simulink model "generic_uservehicle"  (Simulink 7.5)
settings: Solver=ode45  StartTime=0.0  StopTime=inf  RelTol=1e-3
libraries: simulink x6, CarMaker4SL x1
(part 1 of 3)
settings Model: Creator=fh  LastModifiedBy=ml  ExtModeAutoUpdateStatusClock=off
settings DataIOCC: SignalLoggingName=sigsOut
settings OptimizationCC: BooleanDataType=off  InitFltsAndDblsToZero=on
settings DebuggingCC: SaveWithParameterizedLinksMsg=none  SignalResolutionControl=TryResolveAllWithWarning  SolverPrmCheckMsg=none  MultiTaskDSMMsg=warning  MultiTaskCondExecSysMsg=none
settings HardwareCC: TargetUnknown=on
settings RTWCC: IncludeERTFirstTime=on
settings CodeAppCC: MaxIdLength=63
settings GRTTargetCC: TargetFcnLib=ansi_tfl_tmw.mat

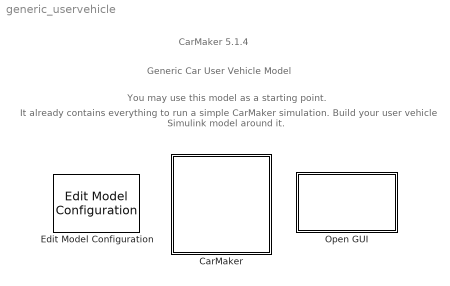
== system generic_uservehicle ==
  note: Generic Car User Vehicle Model
  note: CarMaker 5.1.4
  note: You may use this model as a starting point.
  note: It already contains everything to run a simple CarMaker simulation.
      | Build your user vehicle Simulink model around it.
  CarMaker : Subsystem  TreatAsAtomicUnit=on
      mask Display: image(imread('CarMaker4SLss.bmp'));
  Edit Model Configuration : CarMaker4SL/Edit Model Configuration
  Open GUI : Subsystem  LoadFcn=if ~length(which('cmcmd')), cmenv; end
      settings: OpenFcn=cmblockmagic('gui_fix_display'); CM_Simulink
      mask Display: image(imread('CarMakerGUI.bmp'));

== system generic_uservehicle/CarMaker ==
  CM_FIRST : Subsystem
  CM_LAST : Subsystem
  DrivMan : Subsystem
  Ground : Ground
  Terminator : Terminator
  Vehicle : Subsystem
  VehicleControl : Subsystem
  wires:
  DrivMan/2(DrivMan.Out) -> VehicleControl/2(DrivMan.In)
  DrivMan/1(Sync_Out) -> VehicleControl/1(Sync_In)
  CM_FIRST/2(Env.Misc) -> DrivMan/2(Env.Misc)
  CM_FIRST/1(Sync_Out) -> DrivMan/1(Sync_In)
  CM_LAST/1(Sync_Out) -> Terminator/1
  Ground/1 -> CM_FIRST/1(Sync_In)
  Vehicle/1(Sync_Out) -> CM_LAST/1(Sync_In)
  VehicleControl/1(Sync_Out) -> Vehicle/1(Sync_In)
  VehicleControl/3(VhclCtrl.Steering) -> Vehicle/3(VhclCtrl.Steering)
  VehicleControl/4(Vhcl.Wheel.In) -> Vehicle/4(Vhcl.Wheel.In)
  VehicleControl/5(Vhcl.Misc) -> Vehicle/5(Vhcl.Misc)
  VehicleControl/6(VhclCtrl.Brake) -> Vehicle/6(VhclCtrl.Brake)
  VehicleControl/7(VhclCtrl.PT) -> Vehicle/7(VhclCtrl.PT)
  VehicleControl/2(Vhcl.Model.Source) -> Vehicle/2(Vhcl.Model.Source)

== system generic_uservehicle/Open GUI ==
  S-Function : S-Function  FunctionName=cm_gui  EnableBusSupport=off

== system generic_uservehicle/CarMaker/CM_FIRST ==
  Sync_In : Inport  OutDataType=sfix(16)  OutScaling=2^0
  Bus Creator1 : BusCreator  Inputs=9
  Demux : Demux  Outputs=9
  Environment : S-Function  FunctionName=CM_Sfun  Parameters='Environment'  EnableBusSupport=off
  IoIn : S-Function  FunctionName=CM_Sfun  Parameters='IoIn'  EnableBusSupport=off
  Sync_Out : Outport  OutDataType=sfix(16)  OutScaling=2^0
  Env.Misc : Outport  Port=2  OutDataType=sfix(16)  OutScaling=2^0
  wires:
  Demux/9 -> Bus Creator1/9  "Env WindVel_tot z"
  Demux/8 -> Bus Creator1/8  "Env WindVel_tot y"
  Demux/7 -> Bus Creator1/7  "Env WindVel_tot x"
  Demux/6 -> Bus Creator1/6  "Env SolarRadiation"
  Demux/5 -> Bus Creator1/5  "Env Time"
  Sync_In/1 -> IoIn/1
  IoIn/1 -> Environment/1
  Environment/1 -> Sync_Out/1
  Demux/1 -> Bus Creator1/1  "Env Temperature"
  Demux/2 -> Bus Creator1/2  "Env AirDensity"
  Demux/3 -> Bus Creator1/3  "Env AirPressure"
  Demux/4 -> Bus Creator1/4  "Env AirHumidity"
  Environment/2 -> Demux/1
  Bus Creator1/1 -> Env.Misc/1

== system generic_uservehicle/CarMaker/CM_LAST ==
  Sync_In : Inport  OutDataType=sfix(16)  OutScaling=2^0
  CM_User : S-Function  FunctionName=CM_Sfun  Parameters='CM_User'  EnableBusSupport=off
  IoOut : S-Function  FunctionName=CM_Sfun  Parameters='IoOut'  EnableBusSupport=off
  Sync_Out : Outport  OutDataType=sfix(16)  OutScaling=2^0
  wires:
  IoOut/1 -> Sync_Out/1
  CM_User/1 -> IoOut/1
  Sync_In/1 -> CM_User/1

== system generic_uservehicle/CarMaker/DrivMan ==
  note: There's rarely a reason to override DrivMan signals.
      | Use the VehicleControl interface for this purpose.
  Sync_In : Inport  OutDataType=sfix(16)  OutScaling=2^0
  Env.Misc : Inport  Port=2  OutDataType=sfix(16)  OutScaling=2^0
  BusCreator : BusCreator  Inputs=17
  Demux : Demux  Outputs=17
  DrivMan : S-Function  FunctionName=CM_Sfun  Parameters='DrivMan'  EnableBusSupport=off
  Sync_Out : Outport  OutDataType=sfix(16)  OutScaling=2^0
  DrivMan.Out : Outport  Port=2  OutDataType=sfix(16)  OutScaling=2^0
  wires:
  Demux/17 -> BusCreator/17  "DrivMan Steering Trq"
  Demux/16 -> BusCreator/16  "DrivMan Steering AngAcc"
  Demux/15 -> BusCreator/15  "DrivMan Steering AngVel"
  Demux/14 -> BusCreator/14  "DrivMan Steering Ang"
  Demux/13 -> BusCreator/13  "DrivMan Gas"
  Demux/12 -> BusCreator/12  "DrivMan Clutch"
  Demux/11 -> BusCreator/11  "DrivMan BrakePark"
  Demux/10 -> BusCreator/10  "DrivMan Brake"
  Demux/9 -> BusCreator/9  "DrivMan GearNo"
  Demux/8 -> BusCreator/8  "DrivMan SelectorCtrl"
  Demux/7 -> BusCreator/7  "DrivMan UserSignal4"
  Demux/6 -> BusCreator/6  "DrivMan UserSignal3"
  Demux/5 -> BusCreator/5  "DrivMan UserSignal2"
  Demux/4 -> BusCreator/4  "DrivMan UserSignal1"
  Demux/3 -> BusCreator/3  "DrivMan UserSignal0"
  Demux/2 -> BusCreator/2  "DrivMan Key"
  Demux/1 -> BusCreator/1  "DrivMan SST"
  Env.Misc/1 -> DrivMan/2
  Sync_In/1 -> DrivMan/1
  DrivMan/1 -> Sync_Out/1
  BusCreator/1 -> DrivMan.Out/1
  DrivMan/2 -> Demux/1

== system generic_uservehicle/CarMaker/Vehicle ==
  note: The enabled subsystems allow for simultaneous availability of more than one vehicle.
      | Which one to use will be determined by the vehicle data set of the testrun.
      | If this functionality is not needed, you may simplify your model by using
      | the relevant subsystem of the three as a drop-in replacement for the
      | 'Vehicle' subsystem you're currently looking at, as is done in most of the
      | CarMaker for Simulink example models.
      |
      | PLEASE NOTE: In CarMaker/HIL-ds100x vehicle switching depending on
      | the vehicle data set is not available. To run the user vehicle, the command
      | line option -disablevehicle in the Model Configuration block is required.
  Sync_In : Inport  OutDataType=sfix(16)  OutScaling=2^0
  Vhcl.Model.Source : Inport  Port=2  OutDataType=sfix(16)  OutScaling=2^0
  VhclCtrl.Steering : Inport  Port=3  OutDataType=sfix(16)  OutScaling=2^0
  Vhcl.Wheel.In : Inport  Port=4  OutDataType=sfix(16)  OutScaling=2^0
  Vhcl.Misc : Inport  Port=5  OutDataType=sfix(16)  OutScaling=2^0
  VhclCtrl.Brake : Inport  Port=6  OutDataType=sfix(16)  OutScaling=2^0
  VhclCtrl.PT : Inport  Port=7  OutDataType=sfix(16)  OutScaling=2^0
  IPG Vehicle : Subsystem  TreatAsAtomicUnit=on
  Multiport Switch : MultiPortSwitch  zeroidx=off  InputSameDT=on
  User Vehicle (CM4SL) : Subsystem  TreatAsAtomicUnit=on
  User Vehicle (ModelMgr) : Subsystem  TreatAsAtomicUnit=on
  VehicleSource_BuiltIn : simulink/Logic and Bit Operations/Compare To Constant  SystemSampleTime=-1  relop===  const=1  LogicOutDataTypeMode=boolean  ZeroCross=off
  VehicleSource_CM4SL : simulink/Logic and Bit Operations/Compare To Constant  SystemSampleTime=-1  relop===  const=3  LogicOutDataTypeMode=boolean  ZeroCross=off
  VehicleSource_ModelMgr : simulink/Logic and Bit Operations/Compare To Constant  SystemSampleTime=-1  relop===  const=2  LogicOutDataTypeMode=boolean  ZeroCross=off
  Sync_Out : Outport  OutDataType=sfix(16)  OutScaling=2^0
  wires:
  VhclCtrl.Steering/1 -> IPG Vehicle/3(VhclCtrl.Steering), User Vehicle (ModelMgr)/3(VhclCtrl.Steering), User Vehicle (CM4SL)/3(VhclCtrl.Steering)
  Vhcl.Wheel.In/1 -> IPG Vehicle/4(Vhcl.Wheel.In), User Vehicle (ModelMgr)/4(Vhcl.Wheel.In), User Vehicle (CM4SL)/4(Vhcl.Wheel.In)
  Vhcl.Misc/1 -> IPG Vehicle/5(Vhcl.Misc), User Vehicle (ModelMgr)/5(Vhcl.Misc), User Vehicle (CM4SL)/5(Vhcl.Misc)
  VehicleSource_BuiltIn/1 -> IPG Vehicle/Enable
  VhclCtrl.Brake/1 -> IPG Vehicle/6(VhclCtrl.Brake), User Vehicle (ModelMgr)/6(VhclCtrl.Brake), User Vehicle (CM4SL)/6(VhclCtrl.Brake)
  VhclCtrl.PT/1 -> IPG Vehicle/7(VhclCtrl.PT), User Vehicle (ModelMgr)/7(VhclCtrl.PT), User Vehicle (CM4SL)/7(VhclCtrl.PT)
  Sync_In/1 -> IPG Vehicle/1(Sync_In), User Vehicle (ModelMgr)/1(Sync_In), User Vehicle (CM4SL)/1(Sync_In)
  Vhcl.Model.Source/1 -> VehicleSource_ModelMgr/1, VehicleSource_BuiltIn/1, Multiport Switch/1, IPG Vehicle/2(Vhcl.Model.Source), User Vehicle (ModelMgr)/2(Vhcl.Model.Source), User Vehicle (CM4SL)/2(Vhcl.Model.Source), VehicleSource_CM4SL/1
  VehicleSource_CM4SL/1 -> User Vehicle (CM4SL)/Enable
  VehicleSource_ModelMgr/1 -> User Vehicle (ModelMgr)/Enable
  IPG Vehicle/1(Sync_Out) -> Multiport Switch/2
  User Vehicle (ModelMgr)/1(Sync_Out) -> Multiport Switch/3
  User Vehicle (CM4SL)/1(Sync_Out) -> Multiport Switch/4
  Multiport Switch/1 -> Sync_Out/1

== system generic_uservehicle/CarMaker/VehicleControl ==
  note: <Your model here>
  note: When implementing a vehicle control model,
      | be sure to add '-disablevehiclecontrol' to the command line arguments
      | in the CarMaker Model Configuration block.
      | Otherwise your model will possibly not see the original DrivMan signals
      | on its inputs, but those of a currently activated C-coded vehicle control model instead.
  Sync_In : Inport  OutDataType=sfix(16)  OutScaling=2^0
  DrivMan.In : Inport  Port=2  OutDataType=sfix(16)  OutScaling=2^0
  Bus Creator2 : BusCreator  Inputs=2
  CreateBus Vhcl.Misc : Subsystem
  CreateBus Vhcl.Wheel.In : Subsystem
  CreateBus VhclCtrl : Subsystem
  CreateBus VhclCtrl.PT : Subsystem
  CreateBus VhclCtrl.Steering : Subsystem
  Demux2 : Demux  Outputs=2
  VehicleControl : S-Function  FunctionName=CM_Sfun  Parameters='VehicleControl'  EnableBusSupport=off
  VehicleControlUpd : S-Function  FunctionName=CM_Sfun  Parameters='VehicleControlUpd'  EnableBusSupport=off
  Sync_Out : Outport  OutDataType=sfix(16)  OutScaling=2^0
  Vhcl.Model.Source : Outport  Port=2  OutDataType=sfix(16)  OutScaling=2^0
  VhclCtrl.Steering : Outport  Port=3  OutDataType=sfix(16)  OutScaling=2^0
  Vhcl.Wheel.In : Outport  Port=4  OutDataType=sfix(16)  OutScaling=2^0
  Vhcl.Misc : Outport  Port=5  OutDataType=sfix(16)  OutScaling=2^0
  VhclCtrl.Brake : Outport  Port=6  OutDataType=sfix(16)  OutScaling=2^0
  VhclCtrl.PT : Outport  Port=7  OutDataType=sfix(16)  OutScaling=2^0
  wires:
  CreateBus VhclCtrl/1(Out) -> VehicleControlUpd/2
  VehicleControl/2 -> CreateBus VhclCtrl/1(In)
  VehicleControlUpd/2 -> Vhcl.Model.Source/1
  VehicleControlUpd/4 -> CreateBus Vhcl.Wheel.In/1(In1)
  VehicleControlUpd/5 -> CreateBus Vhcl.Misc/1(In1)
  VehicleControlUpd/6 -> Demux2/1
  VehicleControlUpd/7 -> CreateBus VhclCtrl.PT/1(In1)
  VehicleControlUpd/3 -> CreateBus VhclCtrl.Steering/1(In1)
  CreateBus Vhcl.Misc/1(Out1) -> Vhcl.Misc/1
  CreateBus Vhcl.Wheel.In/1(Out1) -> Vhcl.Wheel.In/1
  DrivMan.In/1 -> VehicleControl/2
  VehicleControl/1 -> VehicleControlUpd/1
  Sync_In/1 -> VehicleControl/1
  CreateBus VhclCtrl.PT/1(Out1) -> VhclCtrl.PT/1
  Bus Creator2/1 -> VhclCtrl.Brake/1
  CreateBus VhclCtrl.Steering/1(Out1) -> VhclCtrl.Steering/1
  VehicleControlUpd/1 -> Sync_Out/1
  Demux2/2 -> Bus Creator2/2  "VhclCtrl BrakePark"
  Demux2/1 -> Bus Creator2/1  "VhclCtrl Brake"

== system generic_uservehicle/CarMaker/Vehicle/IPG Vehicle ==
  Sync_In : Inport  OutDataType=sfix(16)  OutScaling=2^0
  Vhcl.Model.Source : Inport  Port=2  OutDataType=sfix(16)  OutScaling=2^0
  VhclCtrl.Steering : Inport  Port=3  OutDataType=sfix(16)  OutScaling=2^0
  Vhcl.Wheel.In : Inport  Port=4  OutDataType=sfix(16)  OutScaling=2^0
  Vhcl.Misc : Inport  Port=5  OutDataType=sfix(16)  OutScaling=2^0
  VhclCtrl.Brake : Inport  Port=6  OutDataType=sfix(16)  OutScaling=2^0
  VhclCtrl.PT : Inport  Port=7  OutDataType=sfix(16)  OutScaling=2^0
  Enable : EnablePort
  Brake : Subsystem
  CarAndTrailer : Subsystem
  PowerTrain : Subsystem
  Stop Simulation : Stop
  VehicleSource_BuiltIn : simulink/Logic and Bit Operations/Compare To Constant  SystemSampleTime=-1  relop=~=  const=1  LogicOutDataTypeMode=boolean  ZeroCross=off
  Sync_Out : Outport  OutDataType=sfix(16)  OutScaling=2^0
  wires:
  VhclCtrl.PT/1 -> PowerTrain/3(VhclCtrl.PT)
  CarAndTrailer/1(Sync_Out) -> Brake/1(Sync_In)
  CarAndTrailer/2(Brake.IF.In) -> Brake/2(Brake.IF.In)
  VhclCtrl.Brake/1 -> Brake/3(VhclCtrl.Brake)
  PowerTrain/1(Sync_Out) -> Sync_Out/1
  Vhcl.Misc/1 -> CarAndTrailer/4(Vhcl.Misc)
  Vhcl.Wheel.In/1 -> CarAndTrailer/3(Vhcl.Wheel.In)
  VhclCtrl.Steering/1 -> CarAndTrailer/2(VhclCtrl.Steering)
  Sync_In/1 -> CarAndTrailer/1(Sync_In)
  Vhcl.Model.Source/1 -> VehicleSource_BuiltIn/1
  VehicleSource_BuiltIn/1 -> Stop Simulation/1
  Brake/1(Sync_Out) -> PowerTrain/1(Sync_In)
  Brake/2(Vhcl.Wheel.PT) -> PowerTrain/2(Vhcl.Wheel.PT)

== system generic_uservehicle/CarMaker/Vehicle/User Vehicle (CM4SL) ==
  Sync_In : Inport  OutDataType=sfix(16)  OutScaling=2^0
  Vhcl.Model.Source : Inport  Port=2  OutDataType=sfix(16)  OutScaling=2^0
  VhclCtrl.Steering : Inport  Port=3  OutDataType=sfix(16)  OutScaling=2^0
  Vhcl.Wheel.In : Inport  Port=4  OutDataType=sfix(16)  OutScaling=2^0
  Vhcl.Misc : Inport  Port=5  OutDataType=sfix(16)  OutScaling=2^0
  VhclCtrl.Brake : Inport  Port=6  OutDataType=sfix(16)  OutScaling=2^0
  VhclCtrl.PT : Inport  Port=7  OutDataType=sfix(16)  OutScaling=2^0
  Enable : EnablePort
  Brake : Subsystem
  CarAndTrailer : Subsystem
  PowerTrain : Subsystem
  Stop Simulation : Stop
  VehicleSource_CM4SL : simulink/Logic and Bit Operations/Compare To Constant  SystemSampleTime=-1  relop=~=  const=3  LogicOutDataTypeMode=boolean  ZeroCross=off
  Sync_Out : Outport  OutDataType=sfix(16)  OutScaling=2^0
  wires:
  VehicleSource_CM4SL/1 -> Stop Simulation/1
  Sync_In/1 -> CarAndTrailer/1(Sync_In)
  VhclCtrl.Steering/1 -> CarAndTrailer/2(VhclCtrl.Steering)
  Vhcl.Wheel.In/1 -> CarAndTrailer/3(Vhcl.Wheel.In)
  Vhcl.Misc/1 -> CarAndTrailer/4(Vhcl.Misc)
  PowerTrain/1(Sync_Out) -> Sync_Out/1
  VhclCtrl.Brake/1 -> Brake/3(VhclCtrl.Brake)
  CarAndTrailer/2(Brake.IF.In) -> Brake/2(Brake.IF.In)
  CarAndTrailer/1(Sync_Out) -> Brake/1(Sync_In)
  VhclCtrl.PT/1 -> PowerTrain/3(VhclCtrl.PT)
  Vhcl.Model.Source/1 -> VehicleSource_CM4SL/1
  Brake/1(Sync_Out) -> PowerTrain/1(Sync_In)
  Brake/2(Vhcl.Wheel.PT) -> PowerTrain/2(Vhcl.Wheel.PT)

== system generic_uservehicle/CarMaker/Vehicle/User Vehicle (ModelMgr) ==
  Sync_In : Inport  OutDataType=sfix(16)  OutScaling=2^0
  Vhcl.Model.Source : Inport  Port=2  OutDataType=sfix(16)  OutScaling=2^0
  VhclCtrl.Steering : Inport  Port=3  OutDataType=sfix(16)  OutScaling=2^0
  Vhcl.Wheel.In : Inport  Port=4  OutDataType=sfix(16)  OutScaling=2^0
  Vhcl.Misc : Inport  Port=5  OutDataType=sfix(16)  OutScaling=2^0
  VhclCtrl.Brake : Inport  Port=6  OutDataType=sfix(16)  OutScaling=2^0
  VhclCtrl.PT : Inport  Port=7  OutDataType=sfix(16)  OutScaling=2^0
  Enable : EnablePort
  Brake : Subsystem
  CarAndTrailer : Subsystem
  PowerTrain : Subsystem
  Stop Simulation : Stop
  VehicleSource_ModelMgr : simulink/Logic and Bit Operations/Compare To Constant  SystemSampleTime=-1  relop=~=  const=2  LogicOutDataTypeMode=boolean  ZeroCross=off
  Sync_Out : Outport  OutDataType=sfix(16)  OutScaling=2^0
  wires:
  Vhcl.Model.Source/1 -> VehicleSource_ModelMgr/1
  Sync_In/1 -> CarAndTrailer/1(Sync_In)
  VhclCtrl.Brake/1 -> Brake/3(VhclCtrl.Brake)
  VhclCtrl.PT/1 -> PowerTrain/3(VhclCtrl.PT)
  PowerTrain/1(Sync_Out) -> Sync_Out/1
  CarAndTrailer/1(Sync_Out) -> Brake/1(Sync_In)
  CarAndTrailer/2(Brake.IF.In) -> Brake/2(Brake.IF.In)
  Vhcl.Misc/1 -> CarAndTrailer/4(Vhcl.Misc)
  Vhcl.Wheel.In/1 -> CarAndTrailer/3(Vhcl.Wheel.In)
  VhclCtrl.Steering/1 -> CarAndTrailer/2(VhclCtrl.Steering)
  VehicleSource_ModelMgr/1 -> Stop Simulation/1
  Brake/1(Sync_Out) -> PowerTrain/1(Sync_In)
  Brake/2(Vhcl.Wheel.PT) -> PowerTrain/2(Vhcl.Wheel.PT)

== system generic_uservehicle/CarMaker/VehicleControl/CreateBus Vhcl.Misc ==
  In1 : Inport  OutDataType=sfix(16)  OutScaling=2^0
  Bus Creator5 : BusCreator  Inputs=11
  Demux5 : Demux  Outputs=11
  Out1 : Outport  OutDataType=sfix(16)  OutScaling=2^0
  wires:
  Demux5/11 -> Bus Creator5/11  "Vhcl Wind_vel_0 z"
  Demux5/10 -> Bus Creator5/10  "Vhcl Wind_vel_0 y"
  Demux5/9 -> Bus Creator5/9  "Vhcl Wind_vel_0 x"
  Demux5/8 -> Bus Creator5/8  "Vhcl DL2BdyEng y"
  Demux5/7 -> Bus Creator5/7  "Vhcl DL2BdyEng x"
  Demux5/6 -> Bus Creator5/6  "Vhcl TrqDL2Bdy1B z"
  Demux5/5 -> Bus Creator5/5  "Vhcl TrqDL2Bdy1B y"
  Demux5/4 -> Bus Creator5/4  "Vhcl TrqDL2Bdy1B x"
  Demux5/3 -> Bus Creator5/3  "Vhcl Trq_DL2Bdy1 z"
  In1/1 -> Demux5/1
  Bus Creator5/1 -> Out1/1
  Demux5/2 -> Bus Creator5/2  "Vhcl Trq_DL2Bdy1 y"
  Demux5/1 -> Bus Creator5/1  "Vhcl Trq_DL2Bdy1 x"

== system generic_uservehicle/CarMaker/VehicleControl/CreateBus Vhcl.Wheel.In ==
  In1 : Inport  OutDataType=sfix(16)  OutScaling=2^0
  Bus Creator1 : BusCreator  Inputs=12
  Demux1 : Demux  Outputs=12
  Out1 : Outport  OutDataType=sfix(16)  OutScaling=2^0
  wires:
  Demux1/12 -> Bus Creator1/12  "Vhcl Wheel RR rotv"
  Demux1/11 -> Bus Creator1/11  "Vhcl Wheel RR Trq_DL2WC"
  Demux1/10 -> Bus Creator1/10  "Vhcl Wheel RR Trq_B2WC"
  Demux1/9 -> Bus Creator1/9  "Vhcl Wheel RL rotv"
  Demux1/8 -> Bus Creator1/8  "Vhcl Wheel RL Trq_DL2WC"
  Demux1/7 -> Bus Creator1/7  "Vhcl Wheel RL Trq_B2WC"
  Demux1/6 -> Bus Creator1/6  "Vhcl Wheel FR rotv"
  Demux1/5 -> Bus Creator1/5  "Vhcl Wheel FR Trq_DL2WC"
  Demux1/4 -> Bus Creator1/4  "Vhcl Wheel FR Trq_B2WC"
  Demux1/3 -> Bus Creator1/3  "Vhcl Wheel FL rotv"
  In1/1 -> Demux1/1
  Bus Creator1/1 -> Out1/1
  Demux1/2 -> Bus Creator1/2  "Vhcl Wheel FL Trq_DL2WC"
  Demux1/1 -> Bus Creator1/1  "Vhcl Wheel FL Trq_B2WC"

== system generic_uservehicle/CarMaker/VehicleControl/CreateBus VhclCtrl ==
  In : Inport
  BusCreator : BusCreator  Inputs=29
  Demux : Demux  Outputs=29
  Out : Outport
  wires:
  In/1 -> Demux/1
  BusCreator/1 -> Out/1
  Demux/1 -> BusCreator/1  "VhclCtrl SST"
  Demux/2 -> BusCreator/2  "VhclCtrl Key"
  Demux/3 -> BusCreator/3  "VhclCtrl UserSignal0"
  Demux/4 -> BusCreator/4  "VhclCtrl UserSignal1"
  Demux/5 -> BusCreator/5  "VhclCtrl UserSignal2"
  Demux/6 -> BusCreator/6  "VhclCtrl UserSignal3"
  Demux/7 -> BusCreator/7  "VhclCtrl UserSignal4"
  Demux/8 -> BusCreator/8  "VhclCtrl GearNo"
  Demux/9 -> BusCreator/9  "VhclCtrl SelectorCtrl"
  Demux/10 -> BusCreator/10  "VhclCtrl Brake"
  Demux/11 -> BusCreator/11  "VhclCtrl BrakePark"
  Demux/12 -> BusCreator/12  "VhclCtrl Clutch"
  Demux/13 -> BusCreator/13  "VhclCtrl Gas"
  Demux/14 -> BusCreator/14  "VhclCtrl Steering Ang"
  Demux/15 -> BusCreator/15  "VhclCtrl Steering AngVel"
  Demux/16 -> BusCreator/16  "VhclCtrl Steering AngAcc"
  Demux/17 -> BusCreator/17  "VhclCtrl Steering Trq"
  Demux/18 -> BusCreator/18  "VhclCtrl Lights LowBeam"
  Demux/19 -> BusCreator/19  "VhclCtrl Lights HighBeam"
  Demux/20 -> BusCreator/20  "VhclCtrl Lights Daytime"
  Demux/21 -> BusCreator/21  "VhclCtrl Lights ParkL"
  Demux/22 -> BusCreator/22  "VhclCtrl Lights ParkR"
  Demux/23 -> BusCreator/23  "VhclCtrl Lights IndL"
  Demux/24 -> BusCreator/24  "VhclCtrl Lights IndR"
  Demux/25 -> BusCreator/25  "VhclCtrl Lights FogFrontL"
  Demux/26 -> BusCreator/26  "VhclCtrl Lights FogFrontR"
  Demux/27 -> BusCreator/27  "VhclCtrl Lights FogRear"
  Demux/28 -> BusCreator/28  "VhclCtrl Lights Brake"
  Demux/29 -> BusCreator/29  "VhclCtrl Lights Reverse"

== system generic_uservehicle/CarMaker/VehicleControl/CreateBus VhclCtrl.PT ==
  In1 : Inport
  BusCreator : BusCreator  Inputs=11
  Demux : Demux  Outputs=11
  Out1 : Outport
  wires:
  In1/1 -> Demux/1
  BusCreator/1 -> Out1/1
  Demux/1 -> BusCreator/1  "VhclCtrl SST"
  Demux/2 -> BusCreator/2  "VhclCtrl Key"
  Demux/3 -> BusCreator/3  "VhclCtrl UserSignal0"
  Demux/4 -> BusCreator/4  "VhclCtrl UserSignal1"
  Demux/5 -> BusCreator/5  "VhclCtrl UserSignal2"
  Demux/6 -> BusCreator/6  "VhclCtrl UserSignal3"
  Demux/7 -> BusCreator/7  "VhclCtrl UserSignal4"
  Demux/8 -> BusCreator/8  "VhclCtrl GearNo"
  Demux/9 -> BusCreator/9  "VhclCtrl SelectorCtrl"
  Demux/10 -> BusCreator/10  "VhclCtrl Clutch"
  Demux/11 -> BusCreator/11  "VhclCtrl Gas"

== system generic_uservehicle/CarMaker/VehicleControl/CreateBus VhclCtrl.Steering ==
  In1 : Inport  OutDataType=sfix(16)  OutScaling=2^0
  Bus Creator : BusCreator  Inputs=5
  Demux : Demux  Outputs=5
  Out1 : Outport  OutDataType=sfix(16)  OutScaling=2^0
  wires:
  In1/1 -> Demux/1
  Bus Creator/1 -> Out1/1
  Demux/1 -> Bus Creator/1  "VhclCtrl Steering Ang"
  Demux/5 -> Bus Creator/5  "VhclCtrl Steering ByTrq"
  Demux/3 -> Bus Creator/3  "VhclCtrl Steering AngAcc"
  Demux/2 -> Bus Creator/2  "VhclCtrl Steering AngVel"
  Demux/4 -> Bus Creator/4  "VhclCtrl Steering Trq"

== system generic_uservehicle/CarMaker/Vehicle/IPG Vehicle/Brake ==
  note: When replacing the entire braking system,
      | be sure to add '-disablebrake' to the command line arguments
      | in the CarMaker Model Configuration block.
  note: <Your model here>
  Sync_In : Inport  OutDataType=sfix(16)  OutScaling=2^0
  Brake.IF.In : Inport  Port=2  OutDataType=sfix(16)  OutScaling=2^0
  VhclCtrl.Brake : Inport  Port=3  OutDataType=sfix(16)  OutScaling=2^0
  Brake : S-Function  FunctionName=CM_Sfun  Parameters='Brake'  EnableBusSupport=off
  BrakeUpd : S-Function  FunctionName=CM_Sfun  Parameters='BrakeUpd'  EnableBusSupport=off
  BusCreator : BusCreator  Inputs=12
  CreateBus Vhcl.Wheel.PT : Subsystem
  Demux : Demux  Outputs=12
  Sync_Out : Outport  OutDataType=sfix(16)  OutScaling=2^0
  Vhcl.Wheel.PT : Outport  Port=2  OutDataType=sfix(16)  OutScaling=2^0
  wires:
  CreateBus Vhcl.Wheel.PT/1(Out) -> Vhcl.Wheel.PT/1
  BrakeUpd/2 -> CreateBus Vhcl.Wheel.PT/1(In)
  Demux/1 -> BusCreator/1  "Brake IF Trq_WB FL"
  Demux/2 -> BusCreator/2  "Brake IF Trq_WB FR"
  Demux/3 -> BusCreator/3  "Brake IF Trq_WB RL"
  Demux/4 -> BusCreator/4  "Brake IF Trq_WB RR"
  Demux/5 -> BusCreator/5  "Brake IF Trq_PB FL"
  Demux/6 -> BusCreator/6  "Brake IF Trq_PB FR"
  Demux/7 -> BusCreator/7  "Brake IF Trq_PB RL"
  Demux/8 -> BusCreator/8  "Brake IF Trq_PB RR"
  Demux/9 -> BusCreator/9  "Brake IF Trq_Reg_trg FL"
  Demux/10 -> BusCreator/10  "Brake IF Trq_Reg_trg FR"
  Demux/11 -> BusCreator/11  "Brake IF Trq_Reg_trg RL"
  Demux/12 -> BusCreator/12  "Brake IF Trq_Reg_trg RR"
  Sync_In/1 -> Brake/1
  BusCreator/1 -> BrakeUpd/2
  Brake/2 -> Demux/1
  VhclCtrl.Brake/1 -> Brake/3
  Brake.IF.In/1 -> Brake/2
  Brake/1 -> BrakeUpd/1  "Sync"
  BrakeUpd/1 -> Sync_Out/1

== system generic_uservehicle/CarMaker/Vehicle/IPG Vehicle/CarAndTrailer ==
  Sync_In : Inport  OutDataType=sfix(16)  OutScaling=2^0
  VhclCtrl.Steering : Inport  Port=2  OutDataType=sfix(16)  OutScaling=2^0
  Vhcl.Wheel.In : Inport  Port=3  OutDataType=sfix(16)  OutScaling=2^0
  Vhcl.Misc : Inport  Port=4  OutDataType=sfix(16)  OutScaling=2^0
  CarAndTrailerUpd : Subsystem
  Forces : Subsystem
  Ground : Ground
  Kinematics : Subsystem
  Kinetics : Subsystem
  Steering : Subsystem
  Terminator : Terminator
  Terminator1 : Terminator
  Trailer : Subsystem
  Sync_Out : Outport  OutDataType=sfix(16)  OutScaling=2^0
  Brake.IF.In : Outport  Port=2  OutDataType=sfix(16)  OutScaling=2^0
  wires:
  Trailer/9(Car.Hitch.FrcTrq) -> CarAndTrailerUpd/9(Car.Hitch.FrcTrq)
  Trailer/8(Vhcl.Wheel.RR) -> CarAndTrailerUpd/8(Vhcl.Wheel.RR)
  Trailer/7(Vhcl.Wheel.RL) -> CarAndTrailerUpd/7(Vhcl.Wheel.RL)
  Trailer/6(Vhcl.Wheel.FR) -> CarAndTrailerUpd/6(Vhcl.Wheel.FR)
  Trailer/5(Vhcl.Wheel.FL) -> CarAndTrailerUpd/5(Vhcl.Wheel.FL)
  Trailer/4(Vhcl.PoI) -> CarAndTrailerUpd/4(Vhcl.PoI)
  Trailer/3(Vhcl.Motion) -> CarAndTrailerUpd/3(Vhcl.Motion)
  Trailer/2(Vhcl.Steering) -> CarAndTrailerUpd/2(Vhcl.Steering)
  Trailer/1(Sync_Out) -> CarAndTrailerUpd/1(Sync_In)
  CarAndTrailerUpd/2(Brake.IF.In) -> Brake.IF.In/1
  CarAndTrailerUpd/1(Sync_Out) -> Sync_Out/1
  Vhcl.Misc/1 -> Terminator1/1
  Vhcl.Wheel.In/1 -> Terminator/1
  Kinetics/6(WheelCarrier.Misc) -> Trailer/6(WheelCarrier.Misc)
  Kinetics/5(Car.Trq_T2W) -> Trailer/5(Car.Trq_T2W)
  Steering/2(Steer.IF) -> Kinematics/2(Steer.IF)
  Kinetics/4(Car.Fr1) -> Trailer/4(Car.Fr1)
  Kinetics/3(Car.Hitch) -> Trailer/3(Car.Hitch)
  Kinetics/2(Trailer.Load) -> Trailer/2(Trailer.Load)
  VhclCtrl.Steering/1 -> Steering/2(VhclCtrl.Steering)
  Sync_In/1 -> Steering/1(Sync_In)
  Steering/1(Sync_Out) -> Kinematics/1(Sync_In)
  Kinetics/1(Sync_Out) -> Trailer/1(Sync_In)
  Ground/1 -> CarAndTrailerUpd/10(Vhcl.Fr1A)
  Forces/11(FStabi) -> Kinetics/11(FStabi)
  Forces/10(FDamp) -> Kinetics/10(FDamp)
  Forces/9(FSpring) -> Kinetics/9(FSpring)
  Forces/8(TireRR_Out) -> Kinetics/8(TireRR.Out)
  Forces/7(TireRL_Out) -> Kinetics/7(TireRL.Out)
  Forces/6(TireFR_Out) -> Kinetics/6(TireFR.Out)
  Forces/5(TireFL_Out) -> Kinetics/5(TireFL.Out)
  Forces/4(Car.Load) -> Kinetics/4(Car.Load)
  Forces/2(Car.Virtual) -> Kinetics/2(Car.Virtual)
  Kinematics/6(lSpring) -> Forces/6(lSpring)
  Kinematics/7(vDamp) -> Forces/7(vDamp)
  Forces/3(Car.Aero) -> Kinetics/3(Car.Aero)
  Forces/1(Sync_Out) -> Kinetics/1(Sync_In)
  Kinematics/5(TireRR_In) -> Forces/5(TireRR_In)
  Kinematics/4(TireRL_In) -> Forces/4(TireRL_In)
  Kinematics/3(TireFR_In) -> Forces/3(TireFR_In)
  Kinematics/2(TireFL_In) -> Forces/2(TireFL_In)
  Kinematics/1(Sync_Out) -> Forces/1(Sync_In)
  Kinematics/8(lStabi) -> Forces/8(lStabi)
  Forces/12(FBuf) -> Kinetics/12(FBuf)
  Kinematics/9(lBuf) -> Forces/9(lBuf)

== system generic_uservehicle/CarMaker/Vehicle/IPG Vehicle/PowerTrain ==
  note: <Your model here>
  note: When replacing the entire powertrain,
      | be sure to add '-disablepowertrain' to the command line arguments
      | in the CarMaker Model Configuration block.
  Sync_In : Inport  OutDataType=sfix(16)  OutScaling=2^0
  Vhcl.Wheel.PT : Inport  Port=2  OutDataType=sfix(16)  OutScaling=2^0
  VhclCtrl.PT : Inport  Port=3  OutDataType=sfix(16)  OutScaling=2^0
  BusCreator : BusCreator  Inputs=40
  Demux : Demux  Outputs=40
  PowerTrain : S-Function  FunctionName=CM_Sfun  Parameters='PowerTrain'  EnableBusSupport=off
  PowerTrainUpd : S-Function  FunctionName=CM_Sfun  Parameters='PowerTrainUpd'  EnableBusSupport=off
  Sync_Out : Outport  OutDataType=sfix(16)  OutScaling=2^0
  wires:
  Vhcl.Wheel.PT/1 -> PowerTrain/2
  VhclCtrl.PT/1 -> PowerTrain/3
  Demux/40 -> BusCreator/40  "PT IF WRR Trq_BrakeReg_max"
  Demux/39 -> BusCreator/39  "PT IF WRR Trq_BrakeReg"
  Demux/38 -> BusCreator/38  "PT IF WRR Trq_Supp2WC"
  Demux/37 -> BusCreator/37  "PT IF WRR Trq_Drive"
  Demux/36 -> BusCreator/36  "PT IF WRR Trq_B2W"
  Demux/35 -> BusCreator/35  "PT IF WRR rotv"
  Demux/34 -> BusCreator/34  "PT IF WRR rot"
  Demux/33 -> BusCreator/33  "PT IF WRL Trq_BrakeReg_max"
  Demux/32 -> BusCreator/32  "PT IF WRL Trq_BrakeReg"
  Demux/31 -> BusCreator/31  "PT IF WRL Trq_Supp2WC"
  Demux/30 -> BusCreator/30  "PT IF WRL Trq_Drive"
  Demux/29 -> BusCreator/29  "PT IF WRL Trq_B2W"
  Demux/28 -> BusCreator/28  "PT IF WRL rotv"
  Demux/27 -> BusCreator/27  "PT IF WRL rot"
  Demux/26 -> BusCreator/26  "PT IF WFR Trq_BrakeReg_max"
  Demux/25 -> BusCreator/25  "PT IF WFR Trq_BrakeReg"
  Demux/24 -> BusCreator/24  "PT IF WFR Trq_Supp2WC"
  Demux/23 -> BusCreator/23  "PT IF WFR Trq_Drive"
  Demux/22 -> BusCreator/22  "PT IF WFR Trq_B2W"
  Demux/21 -> BusCreator/21  "PT IF WFR rotv"
  Demux/20 -> BusCreator/20  "PT IF WFR rot"
  Demux/19 -> BusCreator/19  "PT IF WFL Trq_BrakeReg_max"
  Demux/18 -> BusCreator/18  "PT IF WFL Trq_BrakeReg"
  Demux/17 -> BusCreator/17  "PT IF WFL Trq_Supp2WC"
  Demux/16 -> BusCreator/16  "PT IF WFL Trq_Drive"
  Demux/15 -> BusCreator/15  "PT IF WFL Trq_B2W"
  Demux/14 -> BusCreator/14  "PT IF WFL rotv"
  Demux/13 -> BusCreator/13  "PT IF WFL rot"
  Demux/12 -> BusCreator/12  "PT IF DL_iDiff_mean"
  Demux/11 -> BusCreator/11  "PT IF Trq_Supp2BdyEng y"
  Demux/10 -> BusCreator/10  "PT IF Trq_Supp2BdyEng x"
  Demux/9 -> BusCreator/9  "PT IF Trq_Supp2Bdy1 z"
  Demux/8 -> BusCreator/8  "PT IF Trq_Supp2Bdy1 y"
  Demux/7 -> BusCreator/7  "PT IF Trq_Supp2Bdy1 x"
  Demux/6 -> BusCreator/6  "PT IF Engine_Trq (EngineControl)"
  Demux/5 -> BusCreator/5  "PT IF Engine_rotv"
  Demux/4 -> BusCreator/4  "PT IF GearNo"
  Demux/3 -> BusCreator/3  "PT IF OperationError"
  Demux/2 -> BusCreator/2  "PT IF OperationState"
  Demux/1 -> BusCreator/1  "PT IF Ignition"
  BusCreator/1 -> PowerTrainUpd/2
  PowerTrain/1 -> PowerTrainUpd/1  "Sync"
  PowerTrainUpd/1 -> Sync_Out/1
  PowerTrain/2 -> Demux/1
  Sync_In/1 -> PowerTrain/1

== system generic_uservehicle/CarMaker/Vehicle/User Vehicle (CM4SL)/Brake ==
  note: When replacing the entire braking system,
      | be sure to add '-disablebrake' to the command line arguments
      | in the CarMaker Model Configuration block.
  note: <Your model here>
  Sync_In : Inport  OutDataType=sfix(16)  OutScaling=2^0
  Brake.IF.In : Inport  Port=2  OutDataType=sfix(16)  OutScaling=2^0
  VhclCtrl.Brake : Inport  Port=3  OutDataType=sfix(16)  OutScaling=2^0
  Brake : S-Function  FunctionName=CM_Sfun  Parameters='Brake'  EnableBusSupport=off
  BrakeUpd : S-Function  FunctionName=CM_Sfun  Parameters='BrakeUpd'  EnableBusSupport=off
  BusCreator : BusCreator  Inputs=12
  CreateBus Vhcl.Wheel.PT : Subsystem
  Demux : Demux  Outputs=12
  Sync_Out : Outport  OutDataType=sfix(16)  OutScaling=2^0
  Vhcl.Wheel.PT : Outport  Port=2  OutDataType=sfix(16)  OutScaling=2^0
  wires:
  CreateBus Vhcl.Wheel.PT/1(Out) -> Vhcl.Wheel.PT/1
  BrakeUpd/2 -> CreateBus Vhcl.Wheel.PT/1(In)
  Demux/1 -> BusCreator/1  "Brake IF Trq_WB FL"
  Demux/2 -> BusCreator/2  "Brake IF Trq_WB FR"
  Demux/3 -> BusCreator/3  "Brake IF Trq_WB RL"
  Demux/4 -> BusCreator/4  "Brake IF Trq_WB RR"
  Demux/5 -> BusCreator/5  "Brake IF Trq_PB FL"
  Demux/6 -> BusCreator/6  "Brake IF Trq_PB FR"
  Demux/7 -> BusCreator/7  "Brake IF Trq_PB RL"
  Demux/8 -> BusCreator/8  "Brake IF Trq_PB RR"
  Demux/9 -> BusCreator/9  "Brake IF Trq_Reg_trg FL"
  Demux/10 -> BusCreator/10  "Brake IF Trq_Reg_trg FR"
  Demux/11 -> BusCreator/11  "Brake IF Trq_Reg_trg RL"
  Demux/12 -> BusCreator/12  "Brake IF Trq_Reg_trg RR"
  Sync_In/1 -> Brake/1
  BusCreator/1 -> BrakeUpd/2
  Brake/2 -> Demux/1
  VhclCtrl.Brake/1 -> Brake/3
  Brake.IF.In/1 -> Brake/2
  Brake/1 -> BrakeUpd/1  "Sync"
  BrakeUpd/1 -> Sync_Out/1

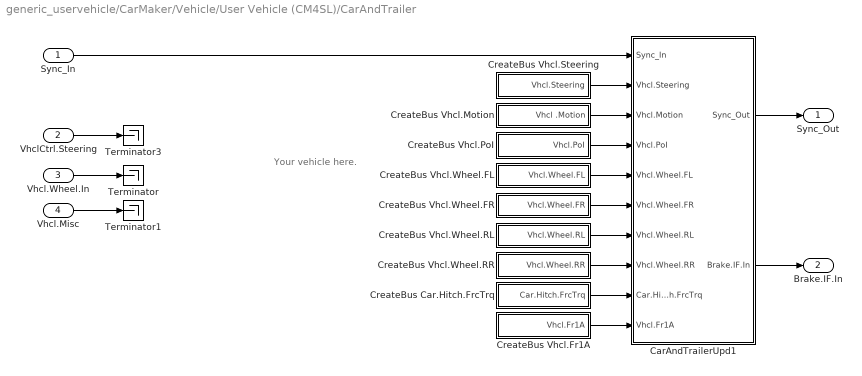
== system generic_uservehicle/CarMaker/Vehicle/User Vehicle (CM4SL)/CarAndTrailer ==
  note: Your vehicle here.
  Sync_In : Inport  OutDataType=sfix(16)  OutScaling=2^0
  VhclCtrl.Steering : Inport  Port=2  OutDataType=sfix(16)  OutScaling=2^0
  Vhcl.Wheel.In : Inport  Port=3  OutDataType=sfix(16)  OutScaling=2^0
  Vhcl.Misc : Inport  Port=4  OutDataType=sfix(16)  OutScaling=2^0
  CarAndTrailerUpd1 : Subsystem
  CreateBus Car.Hitch.FrcTrq : Subsystem
  CreateBus Vhcl.Fr1A : Subsystem
  CreateBus Vhcl.Motion : Subsystem
  CreateBus Vhcl.PoI : Subsystem
  CreateBus Vhcl.Steering : Subsystem
  CreateBus Vhcl.Wheel.FL : Subsystem
  CreateBus Vhcl.Wheel.FR : Subsystem
  CreateBus Vhcl.Wheel.RL : Subsystem
  CreateBus Vhcl.Wheel.RR : Subsystem
  Terminator : Terminator
  Terminator1 : Terminator
  Terminator3 : Terminator
  Sync_Out : Outport  OutDataType=sfix(16)  OutScaling=2^0
  Brake.IF.In : Outport  Port=2  OutDataType=sfix(16)  OutScaling=2^0
  wires:
  CreateBus Vhcl.Fr1A/1(Vhcl.Fr1A) -> CarAndTrailerUpd1/10(Vhcl.Fr1A)
  Sync_In/1 -> CarAndTrailerUpd1/1(Sync_In)
  VhclCtrl.Steering/1 -> Terminator3/1
  Vhcl.Wheel.In/1 -> Terminator/1
  Vhcl.Misc/1 -> Terminator1/1
  CarAndTrailerUpd1/1(Sync_Out) -> Sync_Out/1
  CarAndTrailerUpd1/2(Brake.IF.In) -> Brake.IF.In/1
  CreateBus Car.Hitch.FrcTrq/1(Car.Hitch.FrcTrq) -> CarAndTrailerUpd1/9(Car.Hitch.FrcTrq)
  CreateBus Vhcl.Wheel.RR/1(Vhcl.Wheel.RR) -> CarAndTrailerUpd1/8(Vhcl.Wheel.RR)
  CreateBus Vhcl.Wheel.RL/1(Vhcl.Wheel.RL) -> CarAndTrailerUpd1/7(Vhcl.Wheel.RL)
  CreateBus Vhcl.Wheel.FR/1(Vhcl.Wheel.FR) -> CarAndTrailerUpd1/6(Vhcl.Wheel.FR)
  CreateBus Vhcl.Wheel.FL/1(Vhcl.Wheel.FL) -> CarAndTrailerUpd1/5(Vhcl.Wheel.FL)
  CreateBus Vhcl.PoI/1(Vhcl.PoI) -> CarAndTrailerUpd1/4(Vhcl.PoI)
  CreateBus Vhcl.Motion/1(Vhcl .Motion) -> CarAndTrailerUpd1/3(Vhcl.Motion)
  CreateBus Vhcl.Steering/1(Vhcl.Steering) -> CarAndTrailerUpd1/2(Vhcl.Steering)

== system generic_uservehicle/CarMaker/Vehicle/User Vehicle (CM4SL)/PowerTrain ==
  note: <Your model here>
  note: When replacing the entire powertrain,
      | be sure to add '-disablepowertrain' to the command line arguments
      | in the CarMaker Model Configuration block.
  Sync_In : Inport  OutDataType=sfix(16)  OutScaling=2^0
  Vhcl.Wheel.PT : Inport  Port=2  OutDataType=sfix(16)  OutScaling=2^0
  VhclCtrl.PT : Inport  Port=3  OutDataType=sfix(16)  OutScaling=2^0
  BusCreator : BusCreator  Inputs=40
  Demux : Demux  Outputs=40
  PowerTrain : S-Function  FunctionName=CM_Sfun  Parameters='PowerTrain'  EnableBusSupport=off
  PowerTrainUpd : S-Function  FunctionName=CM_Sfun  Parameters='PowerTrainUpd'  EnableBusSupport=off
  Sync_Out : Outport  OutDataType=sfix(16)  OutScaling=2^0
  wires:
  Vhcl.Wheel.PT/1 -> PowerTrain/2
  VhclCtrl.PT/1 -> PowerTrain/3
  Demux/40 -> BusCreator/40  "PT IF WRR Trq_BrakeReg_max"
  Demux/39 -> BusCreator/39  "PT IF WRR Trq_BrakeReg"
  Demux/38 -> BusCreator/38  "PT IF WRR Trq_Supp2WC"
  Demux/37 -> BusCreator/37  "PT IF WRR Trq_Drive"
  Demux/36 -> BusCreator/36  "PT IF WRR Trq_B2W"
  Demux/35 -> BusCreator/35  "PT IF WRR rotv"
  Demux/34 -> BusCreator/34  "PT IF WRR rot"
  Demux/33 -> BusCreator/33  "PT IF WRL Trq_BrakeReg_max"
  Demux/32 -> BusCreator/32  "PT IF WRL Trq_BrakeReg"
  Demux/31 -> BusCreator/31  "PT IF WRL Trq_Supp2WC"
  Demux/30 -> BusCreator/30  "PT IF WRL Trq_Drive"
  Demux/29 -> BusCreator/29  "PT IF WRL Trq_B2W"
  Demux/28 -> BusCreator/28  "PT IF WRL rotv"
  Demux/27 -> BusCreator/27  "PT IF WRL rot"
  Demux/26 -> BusCreator/26  "PT IF WFR Trq_BrakeReg_max"
  Demux/25 -> BusCreator/25  "PT IF WFR Trq_BrakeReg"
  Demux/24 -> BusCreator/24  "PT IF WFR Trq_Supp2WC"
  Demux/23 -> BusCreator/23  "PT IF WFR Trq_Drive"
  Demux/22 -> BusCreator/22  "PT IF WFR Trq_B2W"
  Demux/21 -> BusCreator/21  "PT IF WFR rotv"
  Demux/20 -> BusCreator/20  "PT IF WFR rot"
  Demux/19 -> BusCreator/19  "PT IF WFL Trq_BrakeReg_max"
  Demux/18 -> BusCreator/18  "PT IF WFL Trq_BrakeReg"
  Demux/17 -> BusCreator/17  "PT IF WFL Trq_Supp2WC"
  Demux/16 -> BusCreator/16  "PT IF WFL Trq_Drive"
  Demux/15 -> BusCreator/15  "PT IF WFL Trq_B2W"
  Demux/14 -> BusCreator/14  "PT IF WFL rotv"
  Demux/13 -> BusCreator/13  "PT IF WFL rot"
  Demux/12 -> BusCreator/12  "PT IF DL_iDiff_mean"
  Demux/11 -> BusCreator/11  "PT IF Trq_Supp2BdyEng y"
  Demux/10 -> BusCreator/10  "PT IF Trq_Supp2BdyEng x"
  Demux/9 -> BusCreator/9  "PT IF Trq_Supp2Bdy1 z"
  Demux/8 -> BusCreator/8  "PT IF Trq_Supp2Bdy1 y"
  Demux/7 -> BusCreator/7  "PT IF Trq_Supp2Bdy1 x"
  Demux/6 -> BusCreator/6  "PT IF Engine_Trq (EngineControl)"
  Demux/5 -> BusCreator/5  "PT IF Engine_rotv"
  Demux/4 -> BusCreator/4  "PT IF GearNo"
  Demux/3 -> BusCreator/3  "PT IF OperationError"
  Demux/2 -> BusCreator/2  "PT IF OperationState"
  Demux/1 -> BusCreator/1  "PT IF Ignition"
  BusCreator/1 -> PowerTrainUpd/2
  PowerTrain/1 -> PowerTrainUpd/1  "Sync"
  PowerTrainUpd/1 -> Sync_Out/1
  PowerTrain/2 -> Demux/1
  Sync_In/1 -> PowerTrain/1

== system generic_uservehicle/CarMaker/Vehicle/User Vehicle (ModelMgr)/Brake ==
  note: When replacing the entire braking system,
      | be sure to add '-disablebrake' to the command line arguments
      | in the CarMaker Model Configuration block.
  note: <Your model here>
  Sync_In : Inport  OutDataType=sfix(16)  OutScaling=2^0
  Brake.IF.In : Inport  Port=2  OutDataType=sfix(16)  OutScaling=2^0
  VhclCtrl.Brake : Inport  Port=3  OutDataType=sfix(16)  OutScaling=2^0
  Brake : S-Function  FunctionName=CM_Sfun  Parameters='Brake'  EnableBusSupport=off
  BrakeUpd : S-Function  FunctionName=CM_Sfun  Parameters='BrakeUpd'  EnableBusSupport=off
  BusCreator : BusCreator  Inputs=12
  CreateBus Vhcl.Wheel.PT : Subsystem
  Demux : Demux  Outputs=12
  Sync_Out : Outport  OutDataType=sfix(16)  OutScaling=2^0
  Vhcl.Wheel.PT : Outport  Port=2  OutDataType=sfix(16)  OutScaling=2^0
  wires:
  CreateBus Vhcl.Wheel.PT/1(Out) -> Vhcl.Wheel.PT/1
  BrakeUpd/2 -> CreateBus Vhcl.Wheel.PT/1(In)
  Demux/1 -> BusCreator/1  "Brake IF Trq_WB FL"
  Demux/2 -> BusCreator/2  "Brake IF Trq_WB FR"
  Demux/3 -> BusCreator/3  "Brake IF Trq_WB RL"
  Demux/4 -> BusCreator/4  "Brake IF Trq_WB RR"
  Demux/5 -> BusCreator/5  "Brake IF Trq_PB FL"
  Demux/6 -> BusCreator/6  "Brake IF Trq_PB FR"
  Demux/7 -> BusCreator/7  "Brake IF Trq_PB RL"
  Demux/8 -> BusCreator/8  "Brake IF Trq_PB RR"
  Demux/9 -> BusCreator/9  "Brake IF Trq_Reg_trg FL"
  Demux/10 -> BusCreator/10  "Brake IF Trq_Reg_trg FR"
  Demux/11 -> BusCreator/11  "Brake IF Trq_Reg_trg RL"
  Demux/12 -> BusCreator/12  "Brake IF Trq_Reg_trg RR"
  Sync_In/1 -> Brake/1
  BusCreator/1 -> BrakeUpd/2
  Brake/2 -> Demux/1
  VhclCtrl.Brake/1 -> Brake/3
  Brake.IF.In/1 -> Brake/2
  Brake/1 -> BrakeUpd/1  "Sync"
  BrakeUpd/1 -> Sync_Out/1

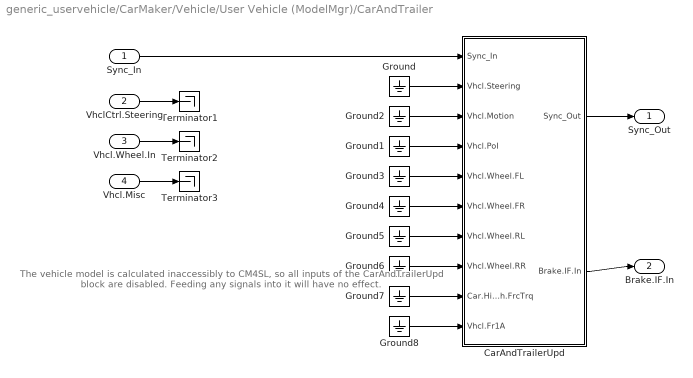
== system generic_uservehicle/CarMaker/Vehicle/User Vehicle (ModelMgr)/CarAndTrailer ==
  note: The vehicle model is calculated inaccessibly to CM4SL,
      | so all inputs of the CarAndTrailerUpd block are disabled.
      | Feeding any signals into it will have no effect.
  Sync_In : Inport  OutDataType=sfix(16)  OutScaling=2^0
  VhclCtrl.Steering : Inport  Port=2  OutDataType=sfix(16)  OutScaling=2^0
  Vhcl.Wheel.In : Inport  Port=3  OutDataType=sfix(16)  OutScaling=2^0
  Vhcl.Misc : Inport  Port=4  OutDataType=sfix(16)  OutScaling=2^0
  CarAndTrailerUpd : Subsystem
  Ground{,1..8} (9 alike) : Ground
  Terminator1 : Terminator
  Terminator2 : Terminator
  Terminator3 : Terminator
  Sync_Out : Outport  OutDataType=sfix(16)  OutScaling=2^0
  Brake.IF.In : Outport  Port=2  OutDataType=sfix(16)  OutScaling=2^0
  wires:
  CarAndTrailerUpd/2(Brake.IF.In) -> Brake.IF.In/1
  CarAndTrailerUpd/1(Sync_Out) -> Sync_Out/1
  Sync_In/1 -> CarAndTrailerUpd/1(Sync_In)
  Ground/1 -> CarAndTrailerUpd/2(Vhcl.Steering)
  Ground2/1 -> CarAndTrailerUpd/3(Vhcl.Motion)
  Ground1/1 -> CarAndTrailerUpd/4(Vhcl.PoI)
  Ground3/1 -> CarAndTrailerUpd/5(Vhcl.Wheel.FL)
  Ground4/1 -> CarAndTrailerUpd/6(Vhcl.Wheel.FR)
  Ground5/1 -> CarAndTrailerUpd/7(Vhcl.Wheel.RL)
  Ground6/1 -> CarAndTrailerUpd/8(Vhcl.Wheel.RR)
  Ground7/1 -> CarAndTrailerUpd/9(Car.Hitch.FrcTrq)
  Ground8/1 -> CarAndTrailerUpd/10(Vhcl.Fr1A)
  VhclCtrl.Steering/1 -> Terminator1/1
  Vhcl.Wheel.In/1 -> Terminator2/1
  Vhcl.Misc/1 -> Terminator3/1

== system generic_uservehicle/CarMaker/Vehicle/User Vehicle (ModelMgr)/PowerTrain ==
  note: <Your model here>
  note: When replacing the entire powertrain,
      | be sure to add '-disablepowertrain' to the command line arguments
      | in the CarMaker Model Configuration block.
  Sync_In : Inport  OutDataType=sfix(16)  OutScaling=2^0
  Vhcl.Wheel.PT : Inport  Port=2  OutDataType=sfix(16)  OutScaling=2^0
  VhclCtrl.PT : Inport  Port=3  OutDataType=sfix(16)  OutScaling=2^0
  BusCreator : BusCreator  Inputs=40
  Demux : Demux  Outputs=40
  PowerTrain : S-Function  FunctionName=CM_Sfun  Parameters='PowerTrain'  EnableBusSupport=off
  PowerTrainUpd : S-Function  FunctionName=CM_Sfun  Parameters='PowerTrainUpd'  EnableBusSupport=off
  Sync_Out : Outport  OutDataType=sfix(16)  OutScaling=2^0
  wires:
  Vhcl.Wheel.PT/1 -> PowerTrain/2
  VhclCtrl.PT/1 -> PowerTrain/3
  Demux/40 -> BusCreator/40  "PT IF WRR Trq_BrakeReg_max"
  Demux/39 -> BusCreator/39  "PT IF WRR Trq_BrakeReg"
  Demux/38 -> BusCreator/38  "PT IF WRR Trq_Supp2WC"
  Demux/37 -> BusCreator/37  "PT IF WRR Trq_Drive"
  Demux/36 -> BusCreator/36  "PT IF WRR Trq_B2W"
  Demux/35 -> BusCreator/35  "PT IF WRR rotv"
  Demux/34 -> BusCreator/34  "PT IF WRR rot"
  Demux/33 -> BusCreator/33  "PT IF WRL Trq_BrakeReg_max"
  Demux/32 -> BusCreator/32  "PT IF WRL Trq_BrakeReg"
  Demux/31 -> BusCreator/31  "PT IF WRL Trq_Supp2WC"
  Demux/30 -> BusCreator/30  "PT IF WRL Trq_Drive"
  Demux/29 -> BusCreator/29  "PT IF WRL Trq_B2W"
  Demux/28 -> BusCreator/28  "PT IF WRL rotv"
  Demux/27 -> BusCreator/27  "PT IF WRL rot"
  Demux/26 -> BusCreator/26  "PT IF WFR Trq_BrakeReg_max"
  Demux/25 -> BusCreator/25  "PT IF WFR Trq_BrakeReg"
  Demux/24 -> BusCreator/24  "PT IF WFR Trq_Supp2WC"
  Demux/23 -> BusCreator/23  "PT IF WFR Trq_Drive"
  Demux/22 -> BusCreator/22  "PT IF WFR Trq_B2W"
  Demux/21 -> BusCreator/21  "PT IF WFR rotv"
  Demux/20 -> BusCreator/20  "PT IF WFR rot"
  Demux/19 -> BusCreator/19  "PT IF WFL Trq_BrakeReg_max"
  Demux/18 -> BusCreator/18  "PT IF WFL Trq_BrakeReg"
  Demux/17 -> BusCreator/17  "PT IF WFL Trq_Supp2WC"
  Demux/16 -> BusCreator/16  "PT IF WFL Trq_Drive"
  Demux/15 -> BusCreator/15  "PT IF WFL Trq_B2W"
  Demux/14 -> BusCreator/14  "PT IF WFL rotv"
  Demux/13 -> BusCreator/13  "PT IF WFL rot"
  Demux/12 -> BusCreator/12  "PT IF DL_iDiff_mean"
  Demux/11 -> BusCreator/11  "PT IF Trq_Supp2BdyEng y"
  Demux/10 -> BusCreator/10  "PT IF Trq_Supp2BdyEng x"
  Demux/9 -> BusCreator/9  "PT IF Trq_Supp2Bdy1 z"
  Demux/8 -> BusCreator/8  "PT IF Trq_Supp2Bdy1 y"
  Demux/7 -> BusCreator/7  "PT IF Trq_Supp2Bdy1 x"
  Demux/6 -> BusCreator/6  "PT IF Engine_Trq (EngineControl)"
  Demux/5 -> BusCreator/5  "PT IF Engine_rotv"
  Demux/4 -> BusCreator/4  "PT IF GearNo"
  Demux/3 -> BusCreator/3  "PT IF OperationError"
  Demux/2 -> BusCreator/2  "PT IF OperationState"
  Demux/1 -> BusCreator/1  "PT IF Ignition"
  BusCreator/1 -> PowerTrainUpd/2
  PowerTrain/1 -> PowerTrainUpd/1  "Sync"
  PowerTrainUpd/1 -> Sync_Out/1
  PowerTrain/2 -> Demux/1
  Sync_In/1 -> PowerTrain/1

== system generic_uservehicle/CarMaker/Vehicle/IPG Vehicle/Brake/CreateBus Vhcl.Wheel.PT ==
  In : Inport
  BusCreator : BusCreator  Inputs=16
  Demux : Demux  Outputs=16
  Out : Outport
  wires:
  In/1 -> Demux/1
  BusCreator/1 -> Out/1
  Demux/1 -> BusCreator/1  "Vhcl Wheel FL Trq_Brake"
  Demux/2 -> BusCreator/2  "Vhcl Wheel FL Trq_BrakeReg_trg"
  Demux/3 -> BusCreator/3  "Vhcl Wheel FL Trq_T2W"
  Demux/4 -> BusCreator/4  "Vhcl Wheel FL WhlBearing"
  Demux/5 -> BusCreator/5  "Vhcl Wheel FR Trq_Brake"
  Demux/6 -> BusCreator/6  "Vhcl Wheel FR Trq_BrakeReg_trg"
  Demux/7 -> BusCreator/7  "Vhcl Wheel FR Trq_T2W"
  Demux/8 -> BusCreator/8  "Vhcl Wheel FR WhlBearing"
  Demux/9 -> BusCreator/9  "Vhcl Wheel RL Trq_Brake"
  Demux/10 -> BusCreator/10  "Vhcl Wheel RL Trq_BrakeReg_trg"
  Demux/11 -> BusCreator/11  "Vhcl Wheel RL Trq_T2W"
  Demux/12 -> BusCreator/12  "Vhcl Wheel RL WhlBearing"
  Demux/13 -> BusCreator/13  "Vhcl Wheel RR Trq_Brake"
  Demux/14 -> BusCreator/14  "Vhcl Wheel RR Trq_BrakeReg_trg"
  Demux/15 -> BusCreator/15  "Vhcl Wheel RR Trq_T2W"
  Demux/16 -> BusCreator/16  "Vhcl Wheel RR WhlBearing"

== system generic_uservehicle/CarMaker/Vehicle/IPG Vehicle/CarAndTrailer/CarAndTrailerUpd ==
  Sync_In : Inport  OutDataType=sfix(16)  OutScaling=2^0
  Vhcl.Steering : Inport  Port=2  OutDataType=sfix(16)  OutScaling=2^0
  Vhcl.Motion : Inport  Port=3  OutDataType=sfix(16)  OutScaling=2^0
  Vhcl.PoI : Inport  Port=4  OutDataType=sfix(16)  OutScaling=2^0
  Vhcl.Wheel.FL : Inport  Port=5  OutDataType=sfix(16)  OutScaling=2^0
  Vhcl.Wheel.FR : Inport  Port=6  OutDataType=sfix(16)  OutScaling=2^0
  Vhcl.Wheel.RL : Inport  Port=7  OutDataType=sfix(16)  OutScaling=2^0
  Vhcl.Wheel.RR : Inport  Port=8  OutDataType=sfix(16)  OutScaling=2^0
  Car.Hitch.FrcTrq : Inport  Port=9  OutDataType=sfix(16)  OutScaling=2^0
  Vhcl.Fr1A : Inport  Port=10  OutDataType=sfix(16)  OutScaling=2^0
  CarAndTrailerUpd : S-Function  FunctionName=CM_Sfun  Parameters='CarAndTrUpd'  EnableBusSupport=off
  CreateBus Brake.IF.In : Subsystem
  Sync_Out : Outport  OutDataType=sfix(16)  OutScaling=2^0
  Brake.IF.In : Outport  Port=2  OutDataType=sfix(16)  OutScaling=2^0
  wires:
  Vhcl.Fr1A/1 -> CarAndTrailerUpd/10  "user vehicle only"
  Vhcl.Steering/1 -> CarAndTrailerUpd/2
  Vhcl.Motion/1 -> CarAndTrailerUpd/3
  Vhcl.PoI/1 -> CarAndTrailerUpd/4
  Vhcl.Wheel.FL/1 -> CarAndTrailerUpd/5
  Vhcl.Wheel.FR/1 -> CarAndTrailerUpd/6
  Car.Hitch.FrcTrq/1 -> CarAndTrailerUpd/9
  Vhcl.Wheel.RR/1 -> CarAndTrailerUpd/8
  Vhcl.Wheel.RL/1 -> CarAndTrailerUpd/7
  CarAndTrailerUpd/2 -> CreateBus Brake.IF.In/1(In)
  CreateBus Brake.IF.In/1(Out) -> Brake.IF.In/1
  CarAndTrailerUpd/1 -> Sync_Out/1
  Sync_In/1 -> CarAndTrailerUpd/1

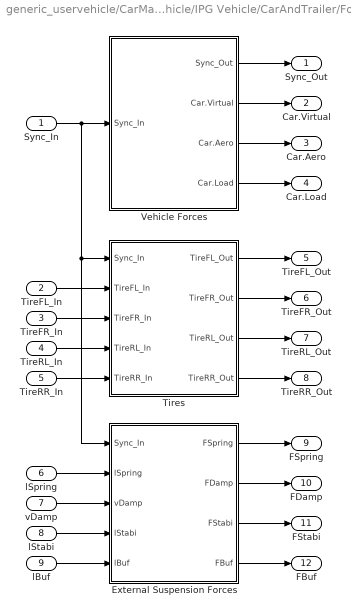
== system generic_uservehicle/CarMaker/Vehicle/IPG Vehicle/CarAndTrailer/Forces ==
  Sync_In : Inport  OutDataType=sfix(16)  OutScaling=2^0
  TireFL_In : Inport  Port=2  OutDataType=sfix(16)  OutScaling=2^0
  TireFR_In : Inport  Port=3  OutDataType=sfix(16)  OutScaling=2^0
  TireRL_In : Inport  Port=4  OutDataType=sfix(16)  OutScaling=2^0
  TireRR_In : Inport  Port=5  OutDataType=sfix(16)  OutScaling=2^0
  lSpring : Inport  Port=6  OutDataType=sfix(16)  OutScaling=2^0
  vDamp : Inport  Port=7  OutDataType=sfix(16)  OutScaling=2^0
  lStabi : Inport  Port=8  OutDataType=sfix(16)  OutScaling=2^0
  lBuf : Inport  Port=9  OutDataType=sfix(16)  OutScaling=2^0
  External Suspension Forces : Subsystem
  Tires : Subsystem
  Vehicle Forces : Subsystem
  Sync_Out : Outport  OutDataType=sfix(16)  OutScaling=2^0
  Car.Virtual : Outport  Port=2  OutDataType=sfix(16)  OutScaling=2^0
  Car.Aero : Outport  Port=3  OutDataType=sfix(16)  OutScaling=2^0
  Car.Load : Outport  Port=4  OutDataType=sfix(16)  OutScaling=2^0
  TireFL_Out : Outport  Port=5  OutDataType=sfix(16)  OutScaling=2^0
  TireFR_Out : Outport  Port=6  OutDataType=sfix(16)  OutScaling=2^0
  TireRL_Out : Outport  Port=7  OutDataType=sfix(16)  OutScaling=2^0
  TireRR_Out : Outport  Port=8  OutDataType=sfix(16)  OutScaling=2^0
  FSpring : Outport  Port=9  OutDataType=sfix(16)  OutScaling=2^0
  FDamp : Outport  Port=10  OutDataType=sfix(16)  OutScaling=2^0
  FStabi : Outport  Port=11  OutDataType=sfix(16)  OutScaling=2^0
  FBuf : Outport  Port=12  OutDataType=sfix(16)  OutScaling=2^0
  wires:
  External Suspension Forces/4(FBuf) -> FBuf/1
  lBuf/1 -> External Suspension Forces/5(lBuf)
  Tires/4(TireRR_Out) -> TireRR_Out/1
  Tires/3(TireRL_Out) -> TireRL_Out/1
  Tires/2(TireFR_Out) -> TireFR_Out/1
  Tires/1(TireFL_Out) -> TireFL_Out/1
  TireRR_In/1 -> Tires/5(TireRR_In)
  TireRL_In/1 -> Tires/4(TireRL_In)
  TireFR_In/1 -> Tires/3(TireFR_In)
  Sync_In/1 -> External Suspension Forces/1(Sync_In), Tires/1(Sync_In), Vehicle Forces/1(Sync_In)
  Vehicle Forces/1(Sync_Out) -> Sync_Out/1
  TireFL_In/1 -> Tires/2(TireFL_In)
  Vehicle Forces/2(Car.Virtual) -> Car.Virtual/1
  Vehicle Forces/3(Car.Aero) -> Car.Aero/1
  Vehicle Forces/4(Car.Load) -> Car.Load/1
  lSpring/1 -> External Suspension Forces/2(lSpring)
  External Suspension Forces/2(FDamp) -> FDamp/1
  vDamp/1 -> External Suspension Forces/3(vDamp)
  lStabi/1 -> External Suspension Forces/4(lStabi)
  External Suspension Forces/3(FStabi) -> FStabi/1
  External Suspension Forces/1(FSpring) -> FSpring/1

== system generic_uservehicle/CarMaker/Vehicle/IPG Vehicle/CarAndTrailer/Kinematics ==
  Sync_In : Inport  OutDataType=sfix(16)  OutScaling=2^0
  Steer.IF : Inport  Port=2  OutDataType=sfix(16)  OutScaling=2^0
  Kinematics : S-Function  FunctionName=CM_Sfun  Parameters='Kinematics'  EnableBusSupport=off
  Sync_Out : Outport  OutDataType=sfix(16)  OutScaling=2^0
  TireFL_In : Outport  Port=2  OutDataType=sfix(16)  OutScaling=2^0
  TireFR_In : Outport  Port=3  OutDataType=sfix(16)  OutScaling=2^0
  TireRL_In : Outport  Port=4  OutDataType=sfix(16)  OutScaling=2^0
  TireRR_In : Outport  Port=5  OutDataType=sfix(16)  OutScaling=2^0
  lSpring : Outport  Port=6  OutDataType=sfix(16)  OutScaling=2^0
  vDamp : Outport  Port=7  OutDataType=sfix(16)  OutScaling=2^0
  lStabi : Outport  Port=8  OutDataType=sfix(16)  OutScaling=2^0
  lBuf : Outport  Port=9  OutDataType=sfix(16)  OutScaling=2^0
  wires:
  Kinematics/9 -> lBuf/1
  Kinematics/8 -> lStabi/1
  Kinematics/2 -> TireFL_In/1
  Kinematics/3 -> TireFR_In/1
  Kinematics/4 -> TireRL_In/1
  Kinematics/5 -> TireRR_In/1
  Kinematics/6 -> lSpring/1
  Kinematics/7 -> vDamp/1
  Sync_In/1 -> Kinematics/1
  Kinematics/1 -> Sync_Out/1
  Steer.IF/1 -> Kinematics/2
